simulink model "main"  (R2020a)
settings: Solver=VariableStepAuto  StartTime=0.0  StopTime=100.0  RelTol=1e-3
values from neighbouring files (symbols this model uses):
  MOI = [ 0.2538 -0.0002  0.0016 ... (first row only)    [gain_calc.m]
libraries: aerolibutil x6, vrlib x2, sharedutil x2, shared6dofsys x2, sharedtransform x2, simulink_extras x2, simulink x2
settings Model: Creator=DanKvist  LastModifiedBy=DanKvist

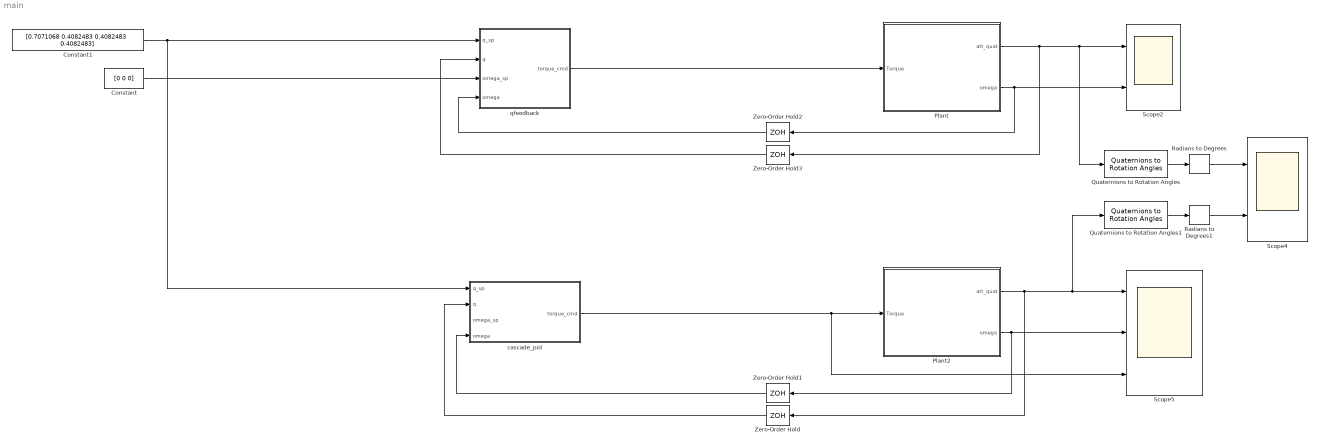
== system main ==
  Constant : Constant  Value=[0 0 0]
  Constant1 : Constant  Value=[0.7071068 0.4082483 0.4082483 0.4082483]
  Plant : Subsystem  mask{Intertia=MOI, omega_0=[0 0 0], q_0=[1 0 0 0]}
      mask prompts: Intertia "System MOI"; omega_0 "Initial rate"; q_0 "Initial att"
  Plant2 : Subsystem  mask{Intertia=MOI, omega_0=[0 0 0], q_0=[1 0 0 0]}
      mask prompts: Intertia "System MOI"; omega_0 "Initial rate"; q_0 "Initial att"
  Quaternions to Rotation Angles : sharedtransform/Quaternions to Rotation Angles  rotationOrder=ZYX  aMode=aMode
      settings: SourceProductBaseCode=AE,PW,MT,VE,VP
  Quaternions to Rotation Angles1 : sharedtransform/Quaternions to Rotation Angles  rotationOrder=ZYX  aMode=aMode
      settings: SourceProductBaseCode=AE,PW,MT,VE,VP
  Radians to Degrees : simulink_extras/Transformations/Radians to Degrees
  Radians to Degrees1 : simulink_extras/Transformations/Radians to Degrees
  Scope2 : Scope  NumInputPorts=2
  Scope4 : Scope  NumInputPorts=2
  Scope5 : Scope  NumInputPorts=3
  Zero-Order Hold{,1..3} (4 alike) : ZeroOrderHold  SampleTime=0.25
  cascade_pid : Subsystem
  qfeedback : Subsystem
  wires:
  Plant/2(omega) -> Scope2/2, Zero-Order Hold2/1
  Plant/1(att_quat) -> Zero-Order Hold3/1, Quaternions to Rotation Angles/1, Scope2/1
  Constant1/1 -> cascade_pid/1(q_sp), qfeedback/1(q_sp)
  qfeedback/1(torque_cmd) -> Plant/1(Torque)
  Plant2/2(omega) -> Zero-Order Hold1/1, Scope5/2
  Plant2/1(att_quat) -> Quaternions to Rotation Angles1/1, Scope5/1, Zero-Order Hold/1
  Constant/1 -> qfeedback/3(omega_sp)
  Quaternions to Rotation Angles/1 -> Radians to Degrees/1
  Radians to Degrees/1 -> Scope4/1
  Quaternions to Rotation Angles1/1 -> Radians to Degrees1/1
  Radians to Degrees1/1 -> Scope4/2
  cascade_pid/1(torque_cmd) -> Plant2/1(Torque), Scope5/3
  Zero-Order Hold/1 -> cascade_pid/2(q)
  Zero-Order Hold1/1 -> cascade_pid/4(omega)
  Zero-Order Hold2/1 -> qfeedback/4(omega)
  Zero-Order Hold3/1 -> qfeedback/2(q)

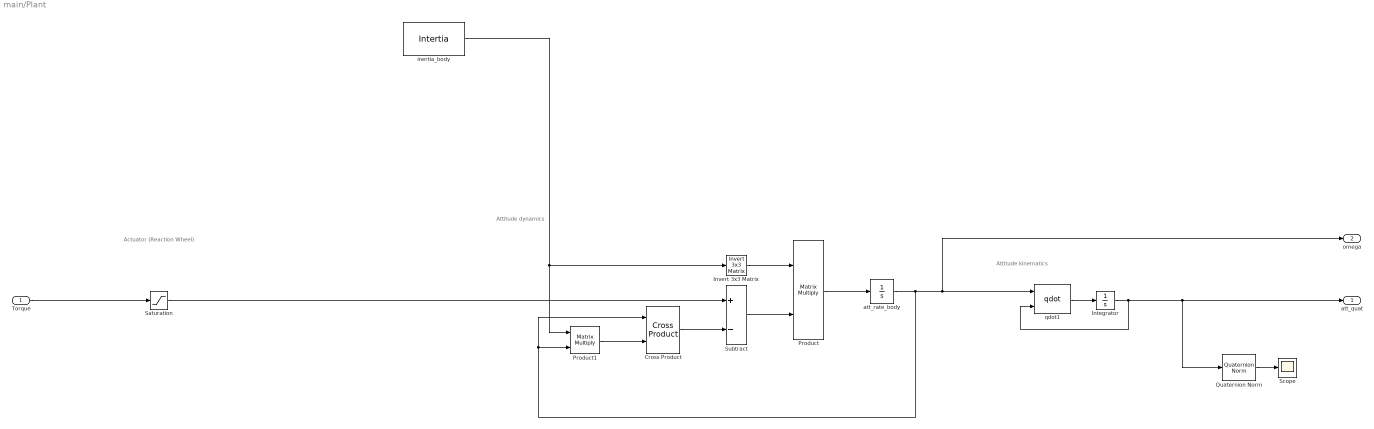
== system main/Plant ==
  note: Actuator (Reaction Wheel)
  note: Attitude kinematics
  note: Attitude dynamics
  Torque : Inport
  Cross Product : vrlib/Utilities/Cross Product
  Integrator : Integrator  InitialCondition=q_0  ContinuousStateAttributes='Attitude'
  Invert 3x3 Matrix : aerolibutil/Invert  3x3 Matrix
  Product : Product  Multiplication=Matrix(*)
  Product1 : Product  Multiplication=Matrix(*)
  Quaternion Norm : sharedutil/Quaternion Norm  aMode=aMode
      settings: SourceProductBaseCode=AE,PW,MT,VE,VP
  Saturation : Saturate  UpperLimit=0.004 * [1 1 1]  LowerLimit=-0.004 * [1 1 1]
  Scope : Scope
  Subtract : Sum  Inputs=+-
  att_rate_body : Integrator  InitialCondition=omega_0  ContinuousStateAttributes='Attitude_Rate'
  inertia_body : Constant  Value=Intertia
  qdot1 : shared6dofsys/qdot  aMode=aMode
      settings: SourceProductBaseCode=AE,PW,MT,VE,VP
  att_quat : Outport
  omega : Outport  Port=2
  wires:
  Cross Product/1 -> Subtract/2
  Invert 3x3 Matrix/1 -> Product/1
  inertia_body/1 -> Product1/1, Invert 3x3 Matrix/1
  Product1/1 -> Cross Product/2
  Integrator/1 -> Quaternion Norm/1, att_quat/1, qdot1/2
  Product/1 -> att_rate_body/1
  att_rate_body/1 -> omega/1, qdot1/1, Product1/2, Cross Product/1
  qdot1/1 -> Integrator/1
  Subtract/1 -> Product/2
  Quaternion Norm/1 -> Scope/1
  Torque/1 -> Saturation/1
  Saturation/1 -> Subtract/1

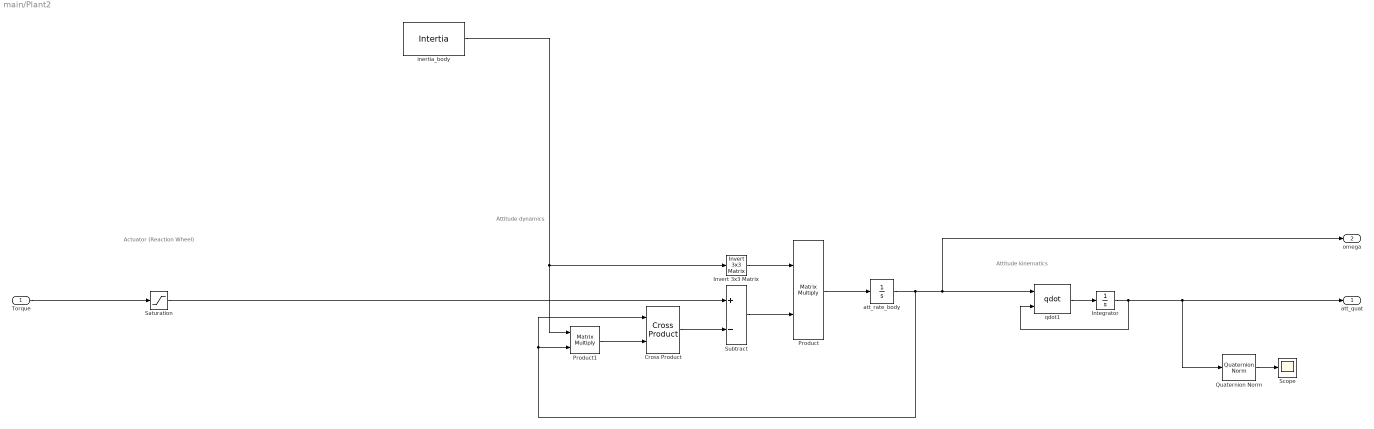
== system main/Plant2 ==
  note: Attitude dynamics
  note: Attitude kinematics
  note: Actuator (Reaction Wheel)
  Torque : Inport
  Cross Product : vrlib/Utilities/Cross Product
  Integrator : Integrator  InitialCondition=q_0  ContinuousStateAttributes='Attitude'
  Invert 3x3 Matrix : aerolibutil/Invert  3x3 Matrix
  Product : Product  Multiplication=Matrix(*)
  Product1 : Product  Multiplication=Matrix(*)
  Quaternion Norm : sharedutil/Quaternion Norm  aMode=aMode
      settings: SourceProductBaseCode=AE,PW,MT,VE,VP
  Saturation : Saturate  UpperLimit=0.004 * [1 1 1]  LowerLimit=-0.004 * [1 1 1]
  Scope : Scope
  Subtract : Sum  Inputs=+-
  att_rate_body : Integrator  InitialCondition=omega_0  ContinuousStateAttributes='Attitude_Rate'
  inertia_body : Constant  Value=Intertia
  qdot1 : shared6dofsys/qdot  aMode=aMode
      settings: SourceProductBaseCode=AE,PW,MT,VE,VP
  att_quat : Outport
  omega : Outport  Port=2
  wires:
  Saturation/1 -> Subtract/1
  Torque/1 -> Saturation/1
  Quaternion Norm/1 -> Scope/1
  Subtract/1 -> Product/2
  qdot1/1 -> Integrator/1
  att_rate_body/1 -> Cross Product/1, Product1/2, qdot1/1, omega/1
  Product/1 -> att_rate_body/1
  Integrator/1 -> qdot1/2, att_quat/1, Quaternion Norm/1
  Product1/1 -> Cross Product/2
  inertia_body/1 -> Invert 3x3 Matrix/1, Product1/1
  Invert 3x3 Matrix/1 -> Product/1
  Cross Product/1 -> Subtract/2

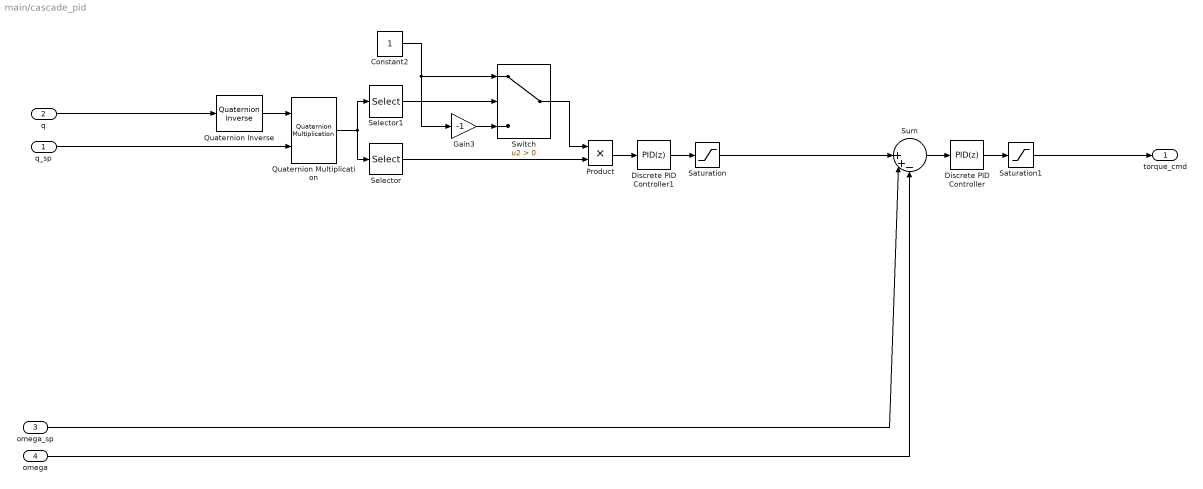
== system main/cascade_pid ==
  q_sp : Inport
  q : Inport  Port=2
  omega_sp : Inport  Port=3
  omega : Inport  Port=4
  Constant2 : Constant
  Discrete PID Controller : simulink/Continuous/PID Controller  Controller=PID  Form=Parallel  TimeDomain=Discrete-time  UseExternalTs=off  SampleTime=-1  IntegratorMethod=Forward Euler  FilterMethod=Forward Euler  ControllerParametersSource=internal  P=[0.2538 0.2128 0.0759]  I=0  D=0  UseFilter=on  N=100  TunerSelectOption=Transfer Function Based (PID Tuner App)  InitialConditionSource=internal  InitialConditionForIntegrator=0  InitialConditionForFilter=0  DifferentiatorICPrevScaledInput=0  ExternalReset=none  TrackingMode=off  Kt=1  LimitOutput=off  UpperSaturationLimit=inf  LowerSaturationLimit=-inf  LinearizeAsGain=off  AntiWindupMode=none  Kb=1  POutMin=[]  POutMax=[]  IOutMin=[]  IOutMax=[]  DOutMin=[]  DOutMax=[]  NOutMin=[]  NOutMax=[]  SumOutMin=[]  SumOutMax=[]  SaturationOutMin=[]  SaturationOutMax=[]  PParamMin=[]  PParamMax=[]  IParamMin=[]  IParamMax=[]  DParamMin=[]  DParamMax=[]  NParamMin=[]  NParamMax=[]  KbParamMin=[]  KbParamMax=[]  KtParamMin=[]  KtParamMax=[]  KbOutMin=[]  KbOutMax=[]  KtOutMin=[]  KtOutMax=[]  IntegratorOutMin=[]  IntegratorOutMax=[]  FilterOutMin=[]  FilterOutMax=[]  SumI1OutMin=[]  SumI1OutMax=[]  SumI2OutMin=[]  SumI2OutMax=[]  SumI3OutMin=[]  SumI3OutMax=[]  SumI4OutMin=[]  SumI4OutMax=[]  SumDOutMin=[]  SumDOutMax=[]  DifferentiatorOutMin=[]  DifferentiatorOutMax=[]  FilterDiffOutCoefMin=[]  FilterDiffOutCoefMax=[]  ReciprocalOutMin=[]  ReciprocalOutMax=[]  SumDenOutMin=[]  SumDenOutMax=[]  SumNumOutMin=[]  SumNumOutMax=[]  DivideOutMin=[]  DivideOutMax=[]  UdiffTsProdOutMin=[]  UdiffTsProdOutMax=[]  NTsProdOutMin=[]  NTsProdOutMax=[]  UintegralTsProdOutMin=[]  UintegralTsProdOutMax=[]  UngainTsProdOutMin=[]  UngainTsProdOutMax=[]  IntegratorContinuousStateAttributes=''  IntegratorStateMustResolveToSignalObject=off  IntegratorRTWStateStorageClass=Auto  FilterContinuousStateAttributes=''  FilterStateMustResolveToSignalObject=off  FilterRTWStateStorageClass=Auto  ParallelPVariant=InternalParameters  IdealPVariant=Disabled  IVariant=InternalParameters  DVariant=InternalParameters  IntegratorVariant=Discrete  SatVariant=Disabled  AWVariant=Passthrough  PCopyVariant=Disabled  TRVariant=Disabled  FdbkBlocksVariant=Forward  IdealPFdbkVariant=Disabled  SatFdbkVariant=Disabled  DerivativeFilterVariant=ForwardEulerFilter  NVariant=InternalParameters  NCopyVariant=Disabled  FilterICVariant=InternalICsFilter  IntegratorICVariant=InternalICs  ExternalResetVariant=Disabled  TRSumVariant=Passthrough  SumFdbkVariant=Disabled  SumVariant=Sum_PID  TsampFilterVariant=InternalTs  TsampNgainVariant=Passthrough  TsampIntegralVariant=Passthrough
  Discrete PID Controller1 : simulink/Continuous/PID Controller  Controller=PID  Form=Parallel  TimeDomain=Discrete-time  UseExternalTs=off  SampleTime=-1  IntegratorMethod=Forward Euler  FilterMethod=Forward Euler  ControllerParametersSource=internal  P=0.5  I=0  D=0  UseFilter=on  N=100  TunerSelectOption=Transfer Function Based (PID Tuner App)  InitialConditionSource=internal  InitialConditionForIntegrator=0  InitialConditionForFilter=0  DifferentiatorICPrevScaledInput=0  ExternalReset=none  TrackingMode=off  Kt=1  LimitOutput=off  UpperSaturationLimit=inf  LowerSaturationLimit=-inf  LinearizeAsGain=off  AntiWindupMode=none  Kb=1  POutMin=[]  POutMax=[]  IOutMin=[]  IOutMax=[]  DOutMin=[]  DOutMax=[]  NOutMin=[]  NOutMax=[]  SumOutMin=[]  SumOutMax=[]  SaturationOutMin=[]  SaturationOutMax=[]  PParamMin=[]  PParamMax=[]  IParamMin=[]  IParamMax=[]  DParamMin=[]  DParamMax=[]  NParamMin=[]  NParamMax=[]  KbParamMin=[]  KbParamMax=[]  KtParamMin=[]  KtParamMax=[]  KbOutMin=[]  KbOutMax=[]  KtOutMin=[]  KtOutMax=[]  IntegratorOutMin=[]  IntegratorOutMax=[]  FilterOutMin=[]  FilterOutMax=[]  SumI1OutMin=[]  SumI1OutMax=[]  SumI2OutMin=[]  SumI2OutMax=[]  SumI3OutMin=[]  SumI3OutMax=[]  SumI4OutMin=[]  SumI4OutMax=[]  SumDOutMin=[]  SumDOutMax=[]  DifferentiatorOutMin=[]  DifferentiatorOutMax=[]  FilterDiffOutCoefMin=[]  FilterDiffOutCoefMax=[]  ReciprocalOutMin=[]  ReciprocalOutMax=[]  SumDenOutMin=[]  SumDenOutMax=[]  SumNumOutMin=[]  SumNumOutMax=[]  DivideOutMin=[]  DivideOutMax=[]  UdiffTsProdOutMin=[]  UdiffTsProdOutMax=[]  NTsProdOutMin=[]  NTsProdOutMax=[]  UintegralTsProdOutMin=[]  UintegralTsProdOutMax=[]  UngainTsProdOutMin=[]  UngainTsProdOutMax=[]  IntegratorContinuousStateAttributes=''  IntegratorStateMustResolveToSignalObject=off  IntegratorRTWStateStorageClass=Auto  FilterContinuousStateAttributes=''  FilterStateMustResolveToSignalObject=off  FilterRTWStateStorageClass=Auto  ParallelPVariant=InternalParameters  IdealPVariant=Disabled  IVariant=InternalParameters  DVariant=InternalParameters  IntegratorVariant=Discrete  SatVariant=Disabled  AWVariant=Passthrough  PCopyVariant=Disabled  TRVariant=Disabled  FdbkBlocksVariant=Forward  IdealPFdbkVariant=Disabled  SatFdbkVariant=Disabled  DerivativeFilterVariant=ForwardEulerFilter  NVariant=InternalParameters  NCopyVariant=Disabled  FilterICVariant=InternalICsFilter  IntegratorICVariant=InternalICs  ExternalResetVariant=Disabled  TRSumVariant=Passthrough  SumFdbkVariant=Disabled  SumVariant=Sum_PID  TsampFilterVariant=InternalTs  TsampNgainVariant=Passthrough  TsampIntegralVariant=Passthrough
  Gain3 : Gain  Gain=-1
  Product : Product
  Quaternion Inverse : aerolibutil/Quaternion Inverse
  Quaternion Multiplication : aerolibutil/Quaternion Multiplication
  Saturation : Saturate  UpperLimit=0.0591 * [1 1 1]  LowerLimit=-0.0591 * [1 1 1]
  Saturation1 : Saturate  UpperLimit=[0.004 0.0034 0.0012]  LowerLimit=-[0.004 0.0034 0.0012]
  Selector : Selector  InputPortWidth=4  IndexOptions=Index vector (dialog)  Indices=[2 3 4]  OutputSizes=1
  Selector1 : Selector  InputPortWidth=4  IndexOptions=Index vector (dialog)  Indices=[1]  OutputSizes=1
  Sum : Sum  Inputs=||++-
  Switch : Switch  Criteria=u2 > Threshold
  torque_cmd : Outport
  wires:
  Gain3/1 -> Switch/3
  Selector1/1 -> Switch/2
  Sum/1 -> Discrete PID Controller/1
  Quaternion Multiplication/1 -> Selector/1, Selector1/1
  Constant2/1 -> Switch/1, Gain3/1
  Quaternion Inverse/1 -> Quaternion Multiplication/1
  omega_sp/1 -> Sum/2
  q_sp/1 -> Quaternion Multiplication/2
  Switch/1 -> Product/1
  Selector/1 -> Product/2
  omega/1 -> Sum/3
  Product/1 -> Discrete PID Controller1/1
  q/1 -> Quaternion Inverse/1
  Discrete PID Controller1/1 -> Saturation/1
  Saturation/1 -> Sum/1
  Discrete PID Controller/1 -> Saturation1/1
  Saturation1/1 -> torque_cmd/1

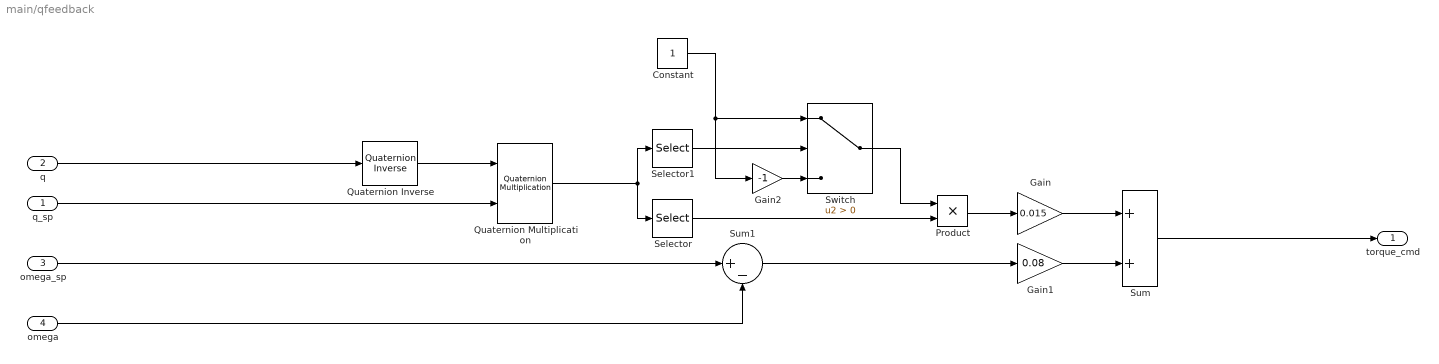
== system main/qfeedback ==
  q_sp : Inport
  q : Inport  Port=2
  omega_sp : Inport  Port=3
  omega : Inport  Port=4
  Constant : Constant
  Gain : Gain  Gain=0.015
  Gain1 : Gain  Gain=0.08
  Gain2 : Gain  Gain=-1
  Product : Product
  Quaternion Inverse : aerolibutil/Quaternion Inverse
  Quaternion Multiplication : aerolibutil/Quaternion Multiplication
  Selector : Selector  InputPortWidth=4  IndexOptions=Index vector (dialog)  Indices=[2 3 4]  OutputSizes=1
  Selector1 : Selector  InputPortWidth=4  IndexOptions=Index vector (dialog)  Indices=[1]  OutputSizes=1
  Sum : Sum
  Sum1 : Sum  Inputs=|+-
  Switch : Switch  Criteria=u2 > Threshold
  torque_cmd : Outport
  wires:
  Selector1/1 -> Switch/2
  Product/1 -> Gain/1
  Selector/1 -> Product/2
  Gain1/1 -> Sum/2
  Quaternion Inverse/1 -> Quaternion Multiplication/1
  omega/1 -> Sum1/2
  Sum1/1 -> Gain1/1
  Quaternion Multiplication/1 -> Selector/1, Selector1/1
  Gain/1 -> Sum/1
  Sum/1 -> torque_cmd/1
  omega_sp/1 -> Sum1/1
  q/1 -> Quaternion Inverse/1
  q_sp/1 -> Quaternion Multiplication/2
  Switch/1 -> Product/1
  Constant/1 -> Gain2/1, Switch/1
  Gain2/1 -> Switch/3
